simulink model "secocnd_order_response"  (R2024b)
settings: Solver=VariableStepAuto  StartTime=0.0  StopTime=10.0  RelTol=1e-3
settings Model: Creator=liaoz  LastModifiedBy=liaoz

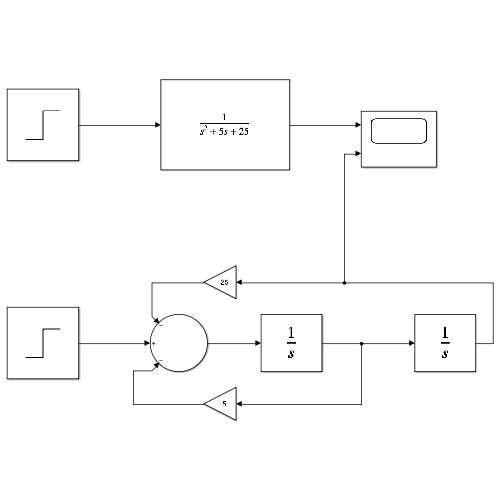
[thumbnail: Simulink's stored preview of the top-level diagram]
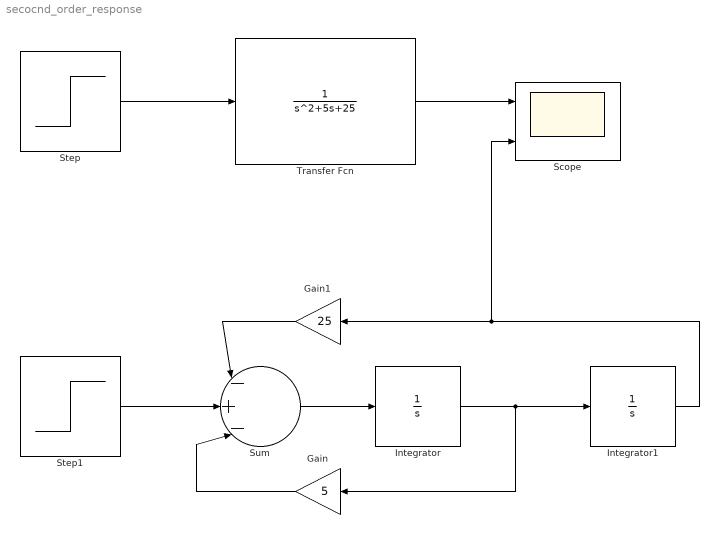
== system secocnd_order_response ==
  Gain : Gain  Gain=5
  Gain1 : Gain  Gain=25
  Integrator : Integrator
  Integrator1 : Integrator
  Scope : Scope  NumInputPorts=2
  Step : Step  Time=0  SampleTime=0
  Step1 : Step  Time=0  SampleTime=0
  Sum : Sum  Inputs=|-+-|
  Transfer Fcn : TransferFcn  Denominator=[1 5 25]
  wires:
  Step/1 -> Transfer Fcn/1
  Transfer Fcn/1 -> Scope/1
  Step1/1 -> Sum/2
  Sum/1 -> Integrator/1
  Integrator/1 -> Gain/1, Integrator1/1
  Gain/1 -> Sum/3
  Integrator1/1 -> Scope/2, Gain1/1
  Gain1/1 -> Sum/1
